simulink model "parcial_3_20240715"  (R2021a)
settings: Solver=VariableStepAuto  StartTime=0.0  StopTime=10.0  RelTol=1e-3
values from neighbouring files (symbols this model uses):
  ue = m*(g*sind(tita)-g*C_r-(1/(2*m))*ro*C_d*a_o*x1e^2)/(alfa_n*T_m*(1-beta*(((alfa_n*x1e)/w_n)-1)^2))    [final_1_20240715.m]
  x1e = 20    [final_1_20240715.m]
  x2e = ue    [final_1_20240715.m]
  x3e = 0    [final_1_20240715.m]
  x4e = 0    [final_1_20240715.m]
libraries: cstblocks x1
settings Model: Creator=frand  LastModifiedBy=frand

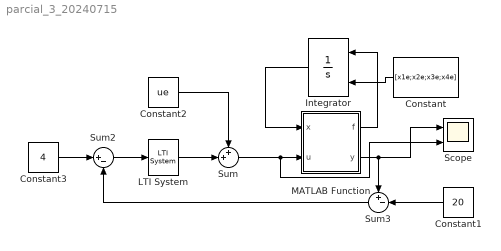
== system parcial_3_20240715 ==
  Constant : Constant  Value=[x1e;x2e;x3e;x4e]
  Constant1 : Constant  Value=20
  Constant2 : Constant  Value=ue
  Constant3 : Constant  Value=4
  Integrator : Integrator  InitialConditionSource=external
  LTI System : cstblocks/LTI System  sys=C_digit  IC=[]
  MATLAB Function : MATLAB Function  TreatAsAtomicUnit=on
  Scope : Scope  NumInputPorts=2
  Sum : Sum  Inputs=++|
  Sum2 : Sum  Inputs=|+-
  Sum3 : Sum  Inputs=+-|
  wires:
  MATLAB Function/2(y) -> Sum3/1, Scope/1
  Sum/1 -> Scope/2, MATLAB Function/2(u)
  MATLAB Function/1(f) -> Integrator/1
  LTI System/1 -> Sum/2
  Sum2/1 -> LTI System/1
  Constant/1 -> Integrator/2
  Sum3/1 -> Sum2/2
  Constant2/1 -> Sum/1
  Constant3/1 -> Sum2/1
  Integrator/1 -> MATLAB Function/1(x)
  Constant1/1 -> Sum3/2

== matlab function parcial_3_20240715/MATLAB Function ==
  data: x input; u input; f output; y output
function [f,y] = fcn(x,u)

m = 1600;
alfa_n = 12;
T_m = 190;
beta = 0.4;
w_n = 420;
w_m = 2*pi;
C_r = 0.01;
ro = 1.3;
C_d = 0.32;
a_o = 2.4;
g = 9.8;
tita = 4;

f1 = (1/m)*(alfa_n*x(2)*T_m*(1-beta*(alfa_n*x(1)/w_n - 1)^2)-m*g*sind(tita)+m*g*C_r+(1/2)*ro*C_d*a_o*x(1)^2);

f2 = x(3);

f3 = x(4);

f4 = -3*w_m*x(4)-3*w_m^2*x(3)-w_m^3*x(2)+w_m^3*u;


f=[f1;f2;f3;f4];

y=x(1);
